simulink model "star_delta"  (R2014a)
settings: Solver=ode23tb  StartTime=0.0  StopTime=0.1  FixedStep=Ts  MaxStep=1e-3  RelTol=1e-4
PreLoadFcn:
  | Ts=2.5e-5;
InitFcn:
  | Ts=2.5e-5;
libraries: powerlib x31
settings Model: Creator=gdudgeon  LastModifiedBy=cosorio
settings DataIOCC: SignalLoggingSaveFormat=ModelDataLogs
settings OptimizationCC: ExpressionDepthLimit=2147483647  InitFltsAndDblsToZero=on
settings DebuggingCC: SaveWithParameterizedLinksMsg=none  UnderspecifiedInitializationDetection=Classic  SignalResolutionControl=TryResolveAllWithWarning  MultiTaskDSMMsg=warning  MultiTaskCondExecSysMsg=none  FcnCallInpInsideContextMsg=UseLocalSettings  StateNameClashWarn=warning
settings RTWCC: IncludeERTFirstTime=on
settings GRTTargetCC: TargetFcnLib=ansi_tfl_tmw.mat  CombineOutputUpdateFcns=off  GRTInterface=on

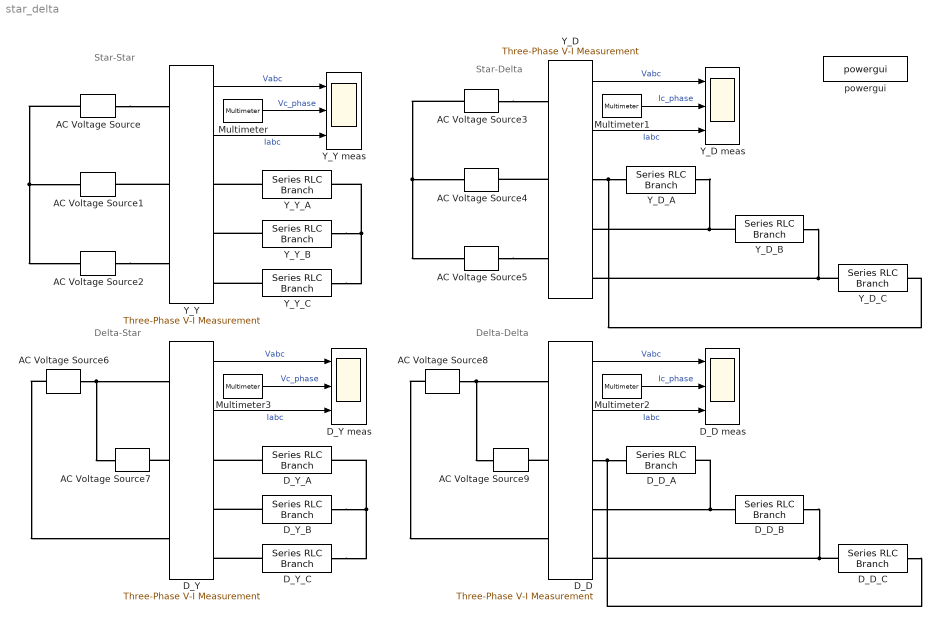
== system star_delta ==
  note: Delta-Delta
  note: Delta-Star
  note: Star-Star
  note: Star-Delta
  AC Voltage Source : powerlib/Electrical Sources/AC Voltage Source  Amplitude=100*sqrt(2)/sqrt(3)  Phase=0  Frequency=60  SampleTime=0  Measurements=None
  AC Voltage Source1 : powerlib/Electrical Sources/AC Voltage Source  Amplitude=100*sqrt(2)/sqrt(3)  Phase=-120  Frequency=60  SampleTime=0  Measurements=None
  AC Voltage Source2 : powerlib/Electrical Sources/AC Voltage Source  Amplitude=100*sqrt(2)/sqrt(3)  Phase=120  Frequency=60  SampleTime=0  Measurements=None
  AC Voltage Source3 : powerlib/Electrical Sources/AC Voltage Source  Amplitude=100*sqrt(2)/sqrt(3)  Phase=0  Frequency=60  SampleTime=0  Measurements=None
  AC Voltage Source4 : powerlib/Electrical Sources/AC Voltage Source  Amplitude=100*sqrt(2)/sqrt(3)  Phase=-120  Frequency=60  SampleTime=0  Measurements=None
  AC Voltage Source5 : powerlib/Electrical Sources/AC Voltage Source  Amplitude=100*sqrt(2)/sqrt(3)  Phase=120  Frequency=60  SampleTime=0  Measurements=None
  AC Voltage Source6 : powerlib/Electrical Sources/AC Voltage Source  Amplitude=100*sqrt(2)  Phase=0  Frequency=60  SampleTime=0  Measurements=None
  AC Voltage Source7 : powerlib/Electrical Sources/AC Voltage Source  Amplitude=100*sqrt(2)  Phase=-120  Frequency=60  SampleTime=0  Measurements=None
  AC Voltage Source8 : powerlib/Electrical Sources/AC Voltage Source  Amplitude=100*sqrt(2)  Phase=0  Frequency=60  SampleTime=0  Measurements=None
  AC Voltage Source9 : powerlib/Electrical Sources/AC Voltage Source  Amplitude=100*sqrt(2)  Phase=-120  Frequency=60  SampleTime=0  Measurements=None
  D_D : powerlib/Measurements/Three-Phase V-I Measurement  VoltageMeasurement=phase-to-phase  SetLabelV=off  LabelV=Vabc  Vpu=off  VpuLL=off  CurrentMeasurement=yes  SetLabelI=off  LabelI=Iabc  Ipu=off  Pbase=100e6  Vbase=500e3  OutputType=Complex  PhasorSimulation=off  PSBequivalent=0
  D_D meas : Scope  NumInputPorts=3
      settings: YMin=-200~-0.1~-0.1  YMax=200~0.1~0.1  SaveName=ScopeData4
  D_D_A : powerlib/Elements/Series RLC Branch  LConnTagsString=__new0  RConnTagsString=__new0  BranchType=RLC  Resistance=1  Inductance=1e-3  SetiL0=off  InitialCurrent=0  Capacitance=1e-6  Setx0=off  InitialVoltage=0  Measurements=None
  D_D_B : powerlib/Elements/Series RLC Branch  LConnTagsString=__new0  RConnTagsString=__new0  BranchType=RLC  Resistance=1  Inductance=1e-3  SetiL0=off  InitialCurrent=0  Capacitance=1e-6  Setx0=off  InitialVoltage=0  Measurements=None
  D_D_C : powerlib/Elements/Series RLC Branch  LConnTagsString=__new0  RConnTagsString=__new0  BranchType=RLC  Resistance=1  Inductance=1e-3  SetiL0=off  InitialCurrent=0  Capacitance=1e-6  Setx0=off  InitialVoltage=0  Measurements=Branch current
  D_Y : powerlib/Measurements/Three-Phase V-I Measurement  VoltageMeasurement=phase-to-phase  SetLabelV=off  LabelV=Vabc  Vpu=off  VpuLL=off  CurrentMeasurement=yes  SetLabelI=off  LabelI=Iabc  Ipu=off  Pbase=100e6  Vbase=500e3  OutputType=Complex  PhasorSimulation=off  PSBequivalent=0
  D_Y meas : Scope  NumInputPorts=3
      settings: YMin=-200~-200~-0.1  YMax=200~200~0.1  SaveName=ScopeData2
  D_Y_A : powerlib/Elements/Series RLC Branch  LConnTagsString=__new0  RConnTagsString=__new0  BranchType=RLC  Resistance=1  Inductance=1e-3  SetiL0=off  InitialCurrent=0  Capacitance=1e-6  Setx0=off  InitialVoltage=0  Measurements=None
  D_Y_B : powerlib/Elements/Series RLC Branch  LConnTagsString=__new0  RConnTagsString=__new0  BranchType=RLC  Resistance=1  Inductance=1e-3  SetiL0=off  InitialCurrent=0  Capacitance=1e-6  Setx0=off  InitialVoltage=0  Measurements=None
  D_Y_C : powerlib/Elements/Series RLC Branch  LConnTagsString=__new0  RConnTagsString=__new0  BranchType=RLC  Resistance=1  Inductance=1e-3  SetiL0=off  InitialCurrent=0  Capacitance=1e-6  Setx0=off  InitialVoltage=0  Measurements=Branch voltage
  Multimeter : powerlib/Measurements/Multimeter  PhasorSimulation=off  OutputType=Complex  sel=2  L=4  Gain=1  yselected={'Ub: Y_Y_C'};  PSBOutputType=1  PSBequivalent=0  AxesSetting=[0,0.1,-100,100]  Display=0  SavedBlockNames=-11
  Multimeter1 : powerlib/Measurements/Multimeter  PhasorSimulation=off  OutputType=Complex  sel=4  L=4  Gain=1  yselected={'Ib: Y_D_C'};  PSBOutputType=1  PSBequivalent=0  AxesSetting=[0,0.1,-100,100]  Display=0  SavedBlockNames=-11
  Multimeter2 : powerlib/Measurements/Multimeter  PhasorSimulation=off  OutputType=Complex  sel=3  L=4  Gain=1  yselected={'Ib: D_D_C'};  PSBOutputType=1  PSBequivalent=0  AxesSetting=[0,0.1,-100,100]  Display=0  SavedBlockNames=-11
  Multimeter3 : powerlib/Measurements/Multimeter  PhasorSimulation=off  OutputType=Complex  sel=1  L=4  Gain=1  yselected={'Ub: D_Y_C'};  PSBOutputType=1  PSBequivalent=0  AxesSetting=[0,0.1,-100,100]  Display=0  SavedBlockNames=-11
  Y_D : powerlib/Measurements/Three-Phase V-I Measurement  VoltageMeasurement=phase-to-phase  SetLabelV=off  LabelV=Vabc  Vpu=off  VpuLL=off  CurrentMeasurement=yes  SetLabelI=off  LabelI=Iabc  Ipu=off  Pbase=100e6  Vbase=500e3  OutputType=Complex  PhasorSimulation=off  PSBequivalent=0
  Y_D meas : Scope  NumInputPorts=3
      settings: YMin=-200~-0.1~-0.1  YMax=200~0.1~0.1
  Y_D_A : powerlib/Elements/Series RLC Branch  LConnTagsString=__new0  RConnTagsString=__new0  BranchType=RLC  Resistance=1  Inductance=1e-3  SetiL0=off  InitialCurrent=0  Capacitance=1e-6  Setx0=off  InitialVoltage=0  Measurements=None
  Y_D_B : powerlib/Elements/Series RLC Branch  LConnTagsString=__new0  RConnTagsString=__new0  BranchType=RLC  Resistance=1  Inductance=1e-3  SetiL0=off  InitialCurrent=0  Capacitance=1e-6  Setx0=off  InitialVoltage=0  Measurements=None
  Y_D_C : powerlib/Elements/Series RLC Branch  LConnTagsString=__new0  RConnTagsString=__new0  BranchType=RLC  Resistance=1  Inductance=1e-3  SetiL0=off  InitialCurrent=0  Capacitance=1e-6  Setx0=off  InitialVoltage=0  Measurements=Branch current
  Y_Y : powerlib/Measurements/Three-Phase V-I Measurement  VoltageMeasurement=phase-to-phase  SetLabelV=off  LabelV=Vabc  Vpu=off  VpuLL=off  CurrentMeasurement=yes  SetLabelI=off  LabelI=Iabc  Ipu=off  Pbase=100e6  Vbase=500e3  OutputType=Complex  PhasorSimulation=off  PSBequivalent=0
  Y_Y meas : Scope  NumInputPorts=3
      settings: YMin=-200~-200~-0.1  YMax=200~200~0.1
  Y_Y_A : powerlib/Elements/Series RLC Branch  LConnTagsString=__new0  RConnTagsString=__new0  BranchType=RLC  Resistance=1  Inductance=1e-3  SetiL0=off  InitialCurrent=0  Capacitance=1e-6  Setx0=off  InitialVoltage=0  Measurements=None
  Y_Y_B : powerlib/Elements/Series RLC Branch  LConnTagsString=__new0  RConnTagsString=__new0  BranchType=RLC  Resistance=1  Inductance=1e-3  SetiL0=off  InitialCurrent=0  Capacitance=1e-6  Setx0=off  InitialVoltage=0  Measurements=None
  Y_Y_C : powerlib/Elements/Series RLC Branch  LConnTagsString=__new0  RConnTagsString=__new0  BranchType=RLC  Resistance=1  Inductance=1e-3  SetiL0=off  InitialCurrent=0  Capacitance=1e-6  Setx0=off  InitialVoltage=0  Measurements=Branch voltage
  powergui : powerlib/powergui  Priority=2  SimulationMode=Continuous  SolverType=Tustin  SampleTime=Ts  frequency=60  SPID=off  DisableSnubberDevices=off  DisableRonSwitches=off  DisableVfSwitches=off  SwTol=0  Interpol=off  DisplayEquations=off  Ts=0  methode=off  frequencyindice=60  Pbase=100e6  ErrMax=1e-4  Iterations=50  UnitsV=kV  UnitsW=MW  FunctionMessages=off  echomessages=off  HookPort=off  EnableUseOfTLC=off  x0status=blocks  RestoreLinks=warning  ResistiveCurrentMeasurement=off  Frange=[0:2:500]  Ylog=off  Xlog=on  ShowGrid=off  save=off  variable=ZData  structure=Iabc2  ZoomFFT=on  StartTime=4  cycles=1  DisplayStyle=1  fundamental=60  FreqAxis=on  MaxFrequency=2000  frequencyindicesteady=1  RmsSteady=1  display=off
  wires:
  Y_Y/1 -> Y_Y meas/1  "Vabc"
  Y_D/1 -> Y_D meas/1  "Vabc"
  Y_D/2 -> Y_D meas/3  "Iabc"
  D_Y/1 -> D_Y meas/1  "Vabc"
  D_Y/2 -> D_Y meas/3  "Iabc"
  D_D/1 -> D_D meas/1  "Vabc"
  D_D/2 -> D_D meas/3  "Iabc"
  Y_Y/2 -> Y_Y meas/3  "Iabc"
  Multimeter/1 -> Y_Y meas/2  "Vc_phase"
  Multimeter1/1 -> Y_D meas/2  "Ic_phase"
  Multimeter2/1 -> D_D meas/2  "Ic_phase"
  Multimeter3/1 -> D_Y meas/2  "Vc_phase"
  connections:
  Y_Y_A/LConn1 -- Y_Y/RConn1
  AC Voltage Source/LConn1 -- AC Voltage Source1/LConn1 -- AC Voltage Source2/LConn1
  AC Voltage Source/RConn1 -- Y_Y/LConn1
  Y_Y/LConn2 -- AC Voltage Source1/RConn1
  AC Voltage Source2/RConn1 -- Y_Y/LConn3
  Y_Y_C/LConn1 -- Y_Y/RConn3
  Y_Y_C/RConn1 -- Y_Y_A/RConn1 -- Y_Y_B/RConn1
  Y_Y_B/LConn1 -- Y_Y/RConn2
  AC Voltage Source3/LConn1 -- AC Voltage Source5/LConn1 -- AC Voltage Source4/LConn1
  Y_D_C/LConn1 -- Y_D_B/RConn1 -- Y_D/RConn3
  Y_D_B/LConn1 -- Y_D_A/RConn1 -- Y_D/RConn2
  AC Voltage Source5/RConn1 -- Y_D/LConn3
  Y_D/LConn2 -- AC Voltage Source4/RConn1
  AC Voltage Source3/RConn1 -- Y_D/LConn1
  Y_D/RConn1 -- Y_D_A/LConn1 -- Y_D_C/RConn1
  AC Voltage Source6/LConn1 -- D_Y/LConn3
  D_Y/LConn2 -- AC Voltage Source7/RConn1
  AC Voltage Source6/RConn1 -- D_Y/LConn1 -- AC Voltage Source7/LConn1
  AC Voltage Source8/RConn1 -- D_D/LConn1 -- AC Voltage Source9/LConn1
  D_D/LConn2 -- AC Voltage Source9/RConn1
  AC Voltage Source8/LConn1 -- D_D/LConn3
  D_Y_C/LConn1 -- D_Y/RConn3
  D_Y_C/RConn1 -- D_Y_B/RConn1 -- D_Y_A/RConn1
  D_Y_B/LConn1 -- D_Y/RConn2
  D_Y_A/LConn1 -- D_Y/RConn1
  D_D_B/RConn1 -- D_D_C/LConn1 -- D_D/RConn3
  D_D/RConn1 -- D_D_A/LConn1 -- D_D_C/RConn1
  D_D/RConn2 -- D_D_B/LConn1 -- D_D_A/RConn1
